simulink model "Transitions1"  (R2020a)
settings: Solver=VariableStepAuto  StartTime=0.0  StopTime=0.1  RelTol=1e-3
settings Model: Creator=BEAR  LastModifiedBy=bzhan
settings DataIOCC: ReturnWorkspaceOutputs=off
settings DebuggingCC: ArithmeticOperatorsInVariantConditions=warning
settings SFSimCC: SimUseLocalCustomCode=off  CustomCodeUndefinedFunction=UseInterfaceOnly
settings RTWCC: RTWUseLocalCustomCode=off

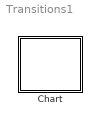
== system Transitions1 ==
  Chart : Stateflow chart  TreatAsAtomicUnit=on

== stateflow chart Transitions1/Chart ==
  settings: updateMethod=DISCRETE  sampleTime=0.1
  state S
    en: f("enS")
    ex: f("exS")
    state A
      en: f("enA")
      ex: f("exA")
    (default) -> A
  state T
    en: f("enT")
    ex: f("exT")
    state B
      en: f("enB")
      ex: f("exB")
    (default) -> B
  (default) -> S
  A -> B : {f("ca")}/{f("ta")}
  data: s function_input
  function f(s):
    | function f(s)
    |   fprintf(s+"\n");
